simulink model "Copy_3_of_canceshi"  (Simulink 8.8)
settings: Solver=ode4  StartTime=0.0  StopTime=inf  FixedStep=0.5  RelTol=1e-3  EnableMultiTasking=on
undefined symbols (not defined in the file or in its folder): bit, Standard
libraries: slrtlib x12, slrtsoftinglib x6, simulink x3
CloseFcn:
  | rtwprivate ssgencode ModelCloseRequest canceshi
settings Model: Creator=Administrator  LastModifiedBy=lenovo  SimulationMode=external
settings SolverCC: EnableConcurrentExecution=on
settings OptimizationCC: BlockReduction=off  OptimizeBlockIOStorage=off  BufferReuse=off  GlobalBufferReuse=off  ExpressionFolding=off  ExpressionDepthLimit=2147483647  LocalBlockOutputs=off  LifeSpan=auto
settings DebuggingCC: SolverPrmCheckMsg=warning
settings HardwareCC: ProdIntDivRoundTo=Zero  ProdEndianess=LittleEndian  ProdLongLongMode=on  ProdHWDeviceType=Generic->32-bit x86 compatible
settings RTWCC: SystemTargetFile=slrt.tlc  TemplateMakefile=slrt_default_tmf  Description=Simulink Real-Time  RTWCompilerOptimization=on

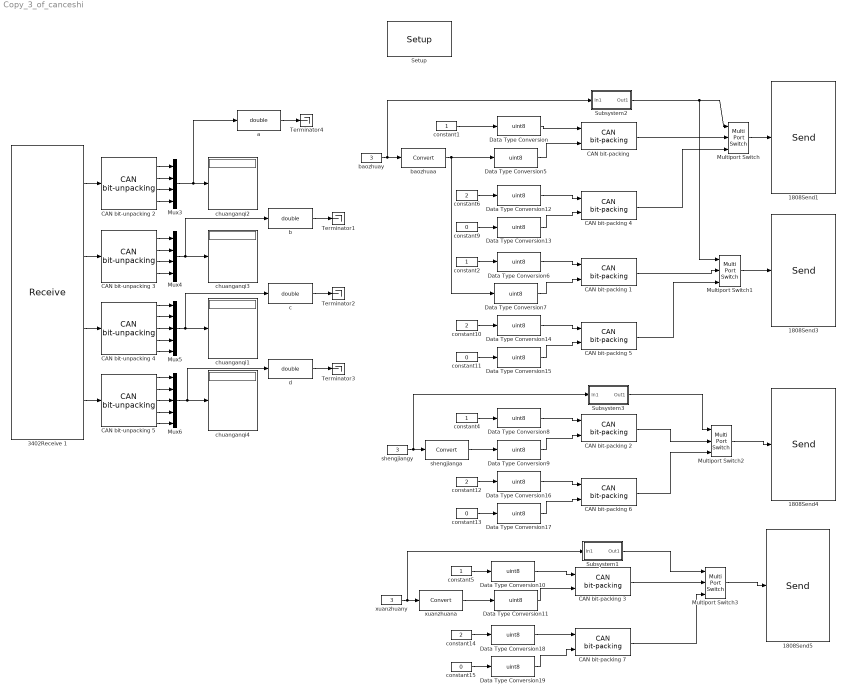
== system Copy_3_of_canceshi ==
  1808Send1 : slrtsoftinglib/CAN-AC2-PCI SJA 1000/Send   board=1  canPort=CAN 1  range=Standard (11-bit)  ids=1  sizes=[8]  output=off  ts=-1  ididx=[0]
  1808Send3 : slrtsoftinglib/CAN-AC2-PCI SJA 1000/Send   board=1  canPort=CAN 2  range=Standard (11-bit)  ids=2  sizes=[8]  output=off  ts=-1  ididx=[0]
  1808Send4 : slrtsoftinglib/CAN-AC2-PCI SJA 1000/Send   board=1  canPort=CAN 2  range=Standard (11-bit)  ids=3  sizes=[8]  output=off  ts=-1  ididx=[1]
  1808Send5 : slrtsoftinglib/CAN-AC2-PCI SJA 1000/Send   board=1  canPort=CAN 2  range=Standard (11-bit)  ids=4  sizes=[8]  output=off  ts=-1  ididx=[2]
  3402Receive 1 : slrtsoftinglib/CAN-AC2-PCI SJA 1000/Receive   board=1  canPort=CAN 2  range=Standard (11-bit)  ids=[1 2 3 4]  lengths=8  output=Data  inten=off  ts=-1  ididx=[0,1,2,3]
  CAN bit-packing {,1..7} (8 alike) : slrtlib/CAN/Utilities/CAN bit-packing   bitpatterns={ [0:7] [8:15] }
  CAN bit-unpacking 2 : slrtlib/CAN/Utilities/CAN bit-unpacking   bitpatterns={ [0:7],[8:15],[16:23],[24:31]}  dtypes={ 'uint8','uint8','uint8','uint8' }
  CAN bit-unpacking 3 : slrtlib/CAN/Utilities/CAN bit-unpacking   bitpatterns={ [0:7],[8:15],[16:23],[24:31]}  dtypes={ 'uint8','uint8','uint8','uint8' }
  CAN bit-unpacking 4 : slrtlib/CAN/Utilities/CAN bit-unpacking   bitpatterns={ [0:7],[8:15],[16:23],[24:31],[32:39]}  dtypes={ 'uint8','uint8','uint8','uint8','uint8' }
  CAN bit-unpacking 5 : slrtlib/CAN/Utilities/CAN bit-unpacking   bitpatterns={ [0:7],[8:15],[16:23],[24:31],[32:39]}  dtypes={ 'uint8','uint8','uint8','uint8','uint8' }
  Data Type Conversion{,5..19} (16 alike) : DataTypeConversion  OutDataTypeStr=uint8
  Multiport Switch{,1..3} (4 alike) : MultiPortSwitch  DataPortOrder=Zero-based contiguous  Inputs=2  zeroidx=on
  Mux3 : Mux
  Mux4 : Mux
  Mux5 : Mux  Inputs=5
  Mux6 : Mux  Inputs=5
  "Setup " : slrtsoftinglib/CAN-AC2-PCI SJA 1000/Setup   board=1  can1bus=Highspeed (ISO 11898)  can1Baudrate=500 kBaud  can1UserBR=[1,1,4,3]  can2bus=Highspeed (ISO 11898)  can2Baudrate=500 kBaud  can2UserBR=[1,1,4,3]  init=[]  term=[]  bus_off_out=off  bus_off_rec=Off  ioBaseAddress=-1
  Subsystem1 : Subsystem
  Subsystem2 : Subsystem
  Subsystem3 : Subsystem
  Terminator{1..4} (4 alike) : Terminator
  a : DataTypeConversion  OutDataTypeStr=double
  b : DataTypeConversion  OutDataTypeStr=double
  baozhuaa : DataTypeConversion
  baozhuay : Constant  Value=3
  c : DataTypeConversion  OutDataTypeStr=double
  chuanganqi{1..4} (4 alike) : Display
  constant{1..2,4..5} (4 alike) : Constant
  constant{6,10,12,14} (4 alike) : Constant  Value=2
  constant{9,11,13,15} (4 alike) : Constant  Value=0
  d : DataTypeConversion  OutDataTypeStr=double
  shengjianga : DataTypeConversion
  shengjiangy : Constant  Value=3
  xuanzhuana : DataTypeConversion
  xuanzhuany : Constant  Value=3
  wires:
  3402Receive 1/1 -> CAN bit-unpacking 2/1
  3402Receive 1/2 -> CAN bit-unpacking 3/1
  3402Receive 1/3 -> CAN bit-unpacking 4/1
  3402Receive 1/4 -> CAN bit-unpacking 5/1
  CAN bit-unpacking 2/1 -> Mux3/1
  CAN bit-unpacking 2/2 -> Mux3/2
  CAN bit-unpacking 2/3 -> Mux3/3
  CAN bit-unpacking 2/4 -> Mux3/4
  CAN bit-unpacking 3/1 -> Mux4/1
  CAN bit-unpacking 3/2 -> Mux4/2
  CAN bit-unpacking 3/3 -> Mux4/3
  CAN bit-unpacking 3/4 -> Mux4/4
  CAN bit-unpacking 4/1 -> Mux5/1
  CAN bit-unpacking 4/2 -> Mux5/2
  CAN bit-unpacking 4/3 -> Mux5/3
  CAN bit-unpacking 4/4 -> Mux5/4
  CAN bit-unpacking 4/5 -> Mux5/5
  CAN bit-unpacking 5/1 -> Mux6/1
  CAN bit-unpacking 5/2 -> Mux6/2
  CAN bit-unpacking 5/3 -> Mux6/3
  CAN bit-unpacking 5/4 -> Mux6/4
  CAN bit-unpacking 5/5 -> Mux6/5
  Mux3/1 -> chuanganqi2/1, a/1
  Mux4/1 -> b/1, chuanganqi3/1
  Mux5/1 -> c/1, chuanganqi1/1
  Mux6/1 -> d/1, chuanganqi4/1
  b/1 -> Terminator1/1
  c/1 -> Terminator2/1
  d/1 -> Terminator3/1
  a/1 -> Terminator4/1
  constant1/1 -> Data Type Conversion/1
  Data Type Conversion/1 -> "CAN bit-packing "/1
  Data Type Conversion5/1 -> "CAN bit-packing "/2
  constant2/1 -> Data Type Conversion6/1
  Data Type Conversion6/1 -> CAN bit-packing 1/1
  Data Type Conversion7/1 -> CAN bit-packing 1/2
  constant4/1 -> Data Type Conversion8/1
  Data Type Conversion8/1 -> CAN bit-packing 2/1
  Data Type Conversion9/1 -> CAN bit-packing 2/2
  constant5/1 -> Data Type Conversion10/1
  Data Type Conversion10/1 -> CAN bit-packing 3/1
  Data Type Conversion11/1 -> CAN bit-packing 3/2
  constant6/1 -> Data Type Conversion12/1
  Data Type Conversion12/1 -> CAN bit-packing 4/1
  Data Type Conversion13/1 -> CAN bit-packing 4/2
  constant9/1 -> Data Type Conversion13/1
  constant10/1 -> Data Type Conversion14/1
  Data Type Conversion14/1 -> CAN bit-packing 5/1
  Data Type Conversion15/1 -> CAN bit-packing 5/2
  constant11/1 -> Data Type Conversion15/1
  constant12/1 -> Data Type Conversion16/1
  Data Type Conversion16/1 -> CAN bit-packing 6/1
  Data Type Conversion17/1 -> CAN bit-packing 6/2
  constant13/1 -> Data Type Conversion17/1
  constant14/1 -> Data Type Conversion18/1
  Data Type Conversion18/1 -> CAN bit-packing 7/1
  Data Type Conversion19/1 -> CAN bit-packing 7/2
  constant15/1 -> Data Type Conversion19/1
  Multiport Switch1/1 -> 1808Send3/1
  baozhuay/1 -> baozhuaa/1, Subsystem2/1(In1)
  shengjiangy/1 -> shengjianga/1, Subsystem3/1(In1)
  shengjianga/1 -> Data Type Conversion9/1
  xuanzhuany/1 -> xuanzhuana/1, Subsystem1/1(In1)
  xuanzhuana/1 -> Data Type Conversion11/1
  Multiport Switch3/1 -> 1808Send5/1
  Multiport Switch/1 -> 1808Send1/1
  Multiport Switch2/1 -> 1808Send4/1
  "CAN bit-packing "/1 -> Multiport Switch/2
  CAN bit-packing 4/1 -> Multiport Switch/3
  CAN bit-packing 1/1 -> Multiport Switch1/2
  CAN bit-packing 5/1 -> Multiport Switch1/3
  CAN bit-packing 2/1 -> Multiport Switch2/2
  CAN bit-packing 6/1 -> Multiport Switch2/3
  CAN bit-packing 3/1 -> Multiport Switch3/2
  CAN bit-packing 7/1 -> Multiport Switch3/3
  baozhuaa/1 -> Data Type Conversion5/1, Data Type Conversion7/1
  Subsystem2/1(Out1) -> Multiport Switch/1, Multiport Switch1/1
  Subsystem3/1(Out1) -> Multiport Switch2/1
  Subsystem1/1(Out1) -> Multiport Switch3/1

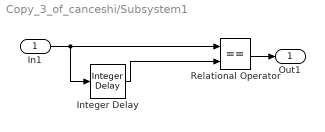
== system Copy_3_of_canceshi/Subsystem1 ==
  In1 : Inport
  Integer Delay : simulink/Discrete/Integer Delay  NumDelays=1  vinit=0.0  samptime=-1
  Relational Operator : RelationalOperator  Operator===  OutDataTypeStr=boolean  RndMeth=Nearest
  Out1 : Outport
  wires:
  Integer Delay/1 -> Relational Operator/2
  In1/1 -> Integer Delay/1, Relational Operator/1
  Relational Operator/1 -> Out1/1

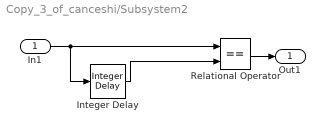
== system Copy_3_of_canceshi/Subsystem2 ==
  In1 : Inport
  Integer Delay : simulink/Discrete/Integer Delay  NumDelays=1  vinit=0.0  samptime=-1
  Relational Operator : RelationalOperator  Operator===  OutDataTypeStr=boolean  RndMeth=Nearest
  Out1 : Outport
  wires:
  Integer Delay/1 -> Relational Operator/2
  In1/1 -> Integer Delay/1, Relational Operator/1
  Relational Operator/1 -> Out1/1

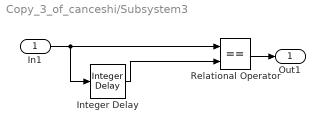
== system Copy_3_of_canceshi/Subsystem3 ==
  In1 : Inport
  Integer Delay : simulink/Discrete/Integer Delay  NumDelays=1  vinit=0.0  samptime=-1
  Relational Operator : RelationalOperator  Operator===  OutDataTypeStr=boolean  RndMeth=Nearest
  Out1 : Outport
  wires:
  Relational Operator/1 -> Out1/1
  In1/1 -> Relational Operator/1, Integer Delay/1
  Integer Delay/1 -> Relational Operator/2
